simulink model "ThreePhaseFullWaveRectifier"  (R2023b)
settings: Solver=VariableStepAuto  StartTime=0.0  StopTime=0.1  RelTol=1e-3
libraries: spsThyristorLib x6, spsMeanLib x4, spsRMSLib x4, spsCurrentMeasurementLib x3, spsSeriesRLCBranchLib x1, spsThreePhaseVIMeasurementLib x1, spsThreePhaseSourceLib x1, spsVoltageMeasurementLib x1, spspowerguiLib x1
settings Model: Creator=Batuhan  LastModifiedBy=yagiz

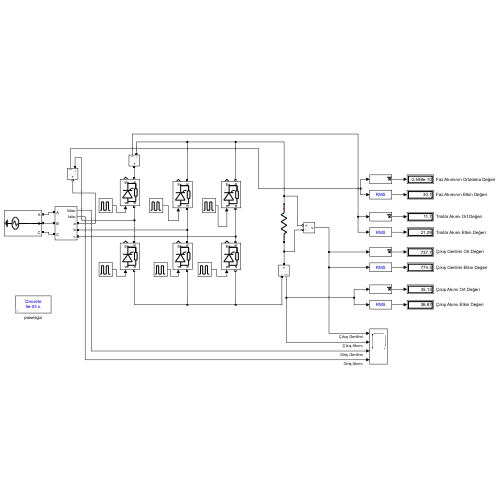
[thumbnail: Simulink's stored preview of the top-level diagram]
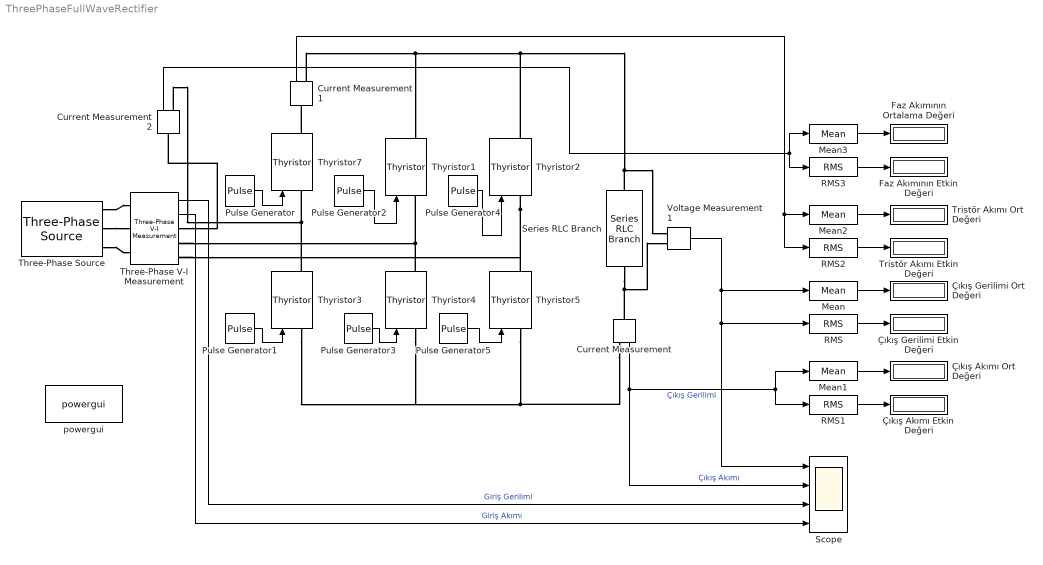
== system ThreePhaseFullWaveRectifier ==
  Current Measurement : spsCurrentMeasurementLib/Current Measurement  PhasorSimulation=off  OutputType=Complex  PSBequivalent=0
  Current Measurement1 : spsCurrentMeasurementLib/Current Measurement  PhasorSimulation=off  OutputType=Complex  PSBequivalent=0
  Current Measurement2 : spsCurrentMeasurementLib/Current Measurement  PhasorSimulation=off  OutputType=Complex  PSBequivalent=0
  Faz Akımının Etkin Değeri : Display
  Faz Akımının Ortalama Değeri : Display
  Mean{,1..3} (4 alike) : spsMeanLib/Mean  Freq=50  Vinit=0  Ts=0
  Pulse Generator : DiscretePulseGenerator  PulseType=Time based  Amplitude=100  Period=0.02  PulseWidth=50  PhaseDelay=75*0.02/360
  Pulse Generator1 : DiscretePulseGenerator  PulseType=Time based  Amplitude=100  Period=0.02  PulseWidth=50  PhaseDelay=255*0.02/360
  Pulse Generator2 : DiscretePulseGenerator  PulseType=Time based  Amplitude=100  Period=0.02  PulseWidth=50  PhaseDelay=195*0.02/360
  Pulse Generator3 : DiscretePulseGenerator  PulseType=Time based  Amplitude=100  Period=0.02  PulseWidth=50  PhaseDelay=15*0.02/360
  Pulse Generator4 : DiscretePulseGenerator  PulseType=Time based  Amplitude=100  Period=0.02  PulseWidth=50  PhaseDelay=315*0.02/360
  Pulse Generator5 : DiscretePulseGenerator  PulseType=Time based  Amplitude=100  Period=0.02  PulseWidth=50  PhaseDelay=135*0.02/360
  RMS{,1..3} (4 alike) : spsRMSLib/RMS  TrueRMS=on  Freq=50  RMSInit=120  Ts=0
  Scope : Scope  NumInputPorts=4
  Series RLC Branch : spsSeriesRLCBranchLib/Series RLC Branch  LConnTagsString=__new0  RConnTagsString=__new0  BranchType=R  Resistance=21  Inductance=1e-3  SetiL0=off  InitialCurrent=0  Capacitance=1e-6  Setx0=off  InitialVoltage=0  Measurements=None
  Three-Phase V-I Measurement : spsThreePhaseVIMeasurementLib/Three-Phase V-I Measurement  VoltageMeasurement=phase-to-ground  SetLabelV=off  LabelV=Vabc  Vpu=off  VpuLL=off  CurrentMeasurement=yes  SetLabelI=off  LabelI=Iabc  Ipu=off  Pbase=100e6  Vbase=500e3  OutputType=Complex  PhasorSimulation=off  PSBequivalent=0
  Three-Phase Source : spsThreePhaseSourceLib/Three-Phase Source  InternalConnection=Yg  VoltagePhases=on  Voltage=452  PhaseAngle=0  Voltage_phases=[452 452 452]  PhaseAngles_phases=[0 -120 +120]  Frequency=50  NonIdealSource=off  SpecifyImpedance=on  Resistance=0.8929  Inductance=16.58e-3  ShortCircuitLevel=100e6  BaseVoltage=25e3  XRratio=7  BusType=swing  Pref=10e3  Qref=0  Prefabc=[10e3, 10e3, 10e3]  Qrefabc=[0, 0, 0]  Qmin=-inf  Qmax=inf
  Thyristor{1..5,7} (6 alike) : spsThyristorLib/Thyristor  Ron=0.001  Lon=0  Vf=0  IC=0  Rs=500  Cs=250e-9  Measurements=on
  Tristör Akımı Etkin Değeri : Display
  Tristör Akımı Ort Değeri : Display
  Voltage Measurement1 : spsVoltageMeasurementLib/Voltage Measurement  PhasorSimulation=off  OutputType=Complex  PSBequivalent=0
  powergui : spspowerguiLib/powergui  Priority=1  SimulationMode=Discrete  SampleTime=50e-6  frequency=60  Iterations=50  frequencyindice=50  Pbase=100e6  ErrMax=1e-4  UnitsV=kV  UnitsW=MW  buscounter=0  FunctionMessages=off  echomessages=off  EnableUseOfTLC=off  CurrentSourceSwitches=off  DisableSnubberDevices=off  DisableRonSwitches=off  DisableVfSwitches=off  DisplayEquations=off  AutomaticDiscreteSolvers=off  SolverType=Tustin/Backward Euler (TBE)  Interpol=off  ExternalGateDelay=off  methode=off  Ts=100  x0status=blocks  SPID=on  SwTol=0  HookPort=off  NonlinearTolerance=1e-4  nMaxIteration=100  ContinueOnMaxIteration=off  RestoreLinks=warning  ResistiveCurrentMeasurement=off  Frange=[0:2:500]  Ylog=off  Xlog=on  ShowGrid=off  save=off  variable=ZData  structure=0  ZoomFFT=off  StartTime=0.0  cycles=1  DisplayStyle=1  fundamental=60  FreqAxis=off  MaxFrequency=1000  frequencyindicesteady=1  RmsSteady=1  display=off
  Çıkış Akımı Etkin Değeri : Display
  Çıkış Akımı Ort Değeri : Display
  Çıkış Gerilimi Etkin Değeri : Display
  Çıkış Gerilimi Ort Değeri : Display
  wires:
  Pulse Generator/1 -> Thyristor7/1
  Pulse Generator1/1 -> Thyristor3/1
  Pulse Generator2/1 -> Thyristor1/1
  Pulse Generator5/1 -> Thyristor5/1
  Pulse Generator3/1 -> Thyristor4/1
  Pulse Generator4/1 -> Thyristor2/1
  Voltage Measurement1/1 -> RMS/1, Scope/1, Mean/1  "Çıkış Gerilimi"
  Current Measurement/1 -> Mean1/1, RMS1/1, Scope/2  "Çıkış Akımı"
  Three-Phase V-I Measurement/1 -> Scope/3  "Giriş Gerilimi"
  Three-Phase V-I Measurement/2 -> Scope/4  "Giriş Akımı"
  Mean/1 -> Çıkış Gerilimi Ort Değeri/1
  RMS/1 -> Çıkış Gerilimi Etkin Değeri/1
  RMS1/1 -> Çıkış Akımı Etkin Değeri/1
  Mean1/1 -> Çıkış Akımı Ort Değeri/1
  RMS2/1 -> Tristör Akımı Etkin Değeri/1
  Mean2/1 -> Tristör Akımı Ort Değeri/1
  Current Measurement1/1 -> Mean2/1, RMS2/1
  RMS3/1 -> Faz Akımının Etkin Değeri/1
  Current Measurement2/1 -> RMS3/1, Mean3/1
  Mean3/1 -> Faz Akımının Ortalama Değeri/1
  connections:
  Three-Phase V-I Measurement/RConn1 -- Current Measurement2/LConn1
  Series RLC Branch/RConn1 -- Current Measurement/LConn1 -- Voltage Measurement1/LConn2
  Three-Phase V-I Measurement/RConn2 -- Thyristor4/RConn1 -- Thyristor1/LConn1
  Thyristor2/LConn1 -- Thyristor5/RConn1 -- Three-Phase V-I Measurement/RConn3
  Three-Phase Source/RConn1 -- Three-Phase V-I Measurement/LConn1
  Three-Phase Source/RConn2 -- Three-Phase V-I Measurement/LConn2
  Three-Phase Source/RConn3 -- Three-Phase V-I Measurement/LConn3
  Thyristor7/RConn1 -- Current Measurement1/LConn1
  Current Measurement1/RConn1 -- Series RLC Branch/LConn1 -- Voltage Measurement1/LConn1 -- Thyristor2/RConn1 -- Thyristor1/RConn1
  Thyristor3/LConn1 -- Thyristor4/LConn1 -- Thyristor5/LConn1 -- Current Measurement/RConn1
  Thyristor3/RConn1 -- Current Measurement2/RConn1 -- Thyristor7/LConn1
